simulink model "mchp_acim_dsPIC33A"  (R2025b)
settings: Solver=FixedStepDiscrete  StartTime=0.0  StopTime=25  FixedStep=Ts  RelTol=1e-3  EnableMultiTasking=on
values from neighbouring files (symbols this model uses):
  dataType = 'single'    [mchp_acim_foc_dsPIC33A_data.m]
  PWM_frequency = 20e3    (= 20000)    [mchp_acim_foc_dsPIC33A_data.m]
  PWM_frequency_mc = PWM_frequency    (= 20000)    [mchp_acim_foc_dsPIC33A_data.m]
  SpeedFilterCutoff = 40    [mchp_acim_foc_dsPIC33A_data.m]
  Ts = T_pwm    (= 5e-05)    [mchp_acim_foc_dsPIC33A_data.m]
  Ts_mc = T_pwm_mc    (= 5e-05)    [mchp_acim_foc_dsPIC33A_data.m]
  Ts_motor = T_pwm_mc    (= 5e-05)    [mchp_acim_foc_dsPIC33A_data.m]
  Ts_serialIn = 100e-3    (= 0.1)    [mchp_acim_foc_dsPIC33A_data.m]
undefined symbols (not defined in the file or in its folder): A0, A4, acim, ADC, appState, B0, C10, C11, C6, C7, C8, CS_param, D11, D12, DiscIntNeverNeededParam, estim_pll, estim_qei, inverter, Max, MaxPer, ms, NumBits1, NumBits2, P1, P17, P20, P39, P40, P41, P43, P44, P60, P61, PI_params_SI, Pin, PWM4_Trg1, Resol, s, target, us, VmaxPhase
libraries: simulink x47, MCHP_Blockset x24, mcbcontrolslib x5, mcbeeMathTransformLib x4, slpidlib x4, svdutilitieslib x1, autolibim x1, mcbplantlib x1
(part 3 of 6)

== system mchp_acim_dsPIC33A/Subsystem ==
  Control mode : Constant  OutDataTypeStr=single
  DC bus compensation : Constant  OutDataTypeStr=single  SampleTime=-1
  Data Store Write : DataStoreWrite  DataStoreName=ControlMode  IndexOptions=Index vector (dialog)  Indices=1  OutputSizes=1
  Data Store Write1 : DataStoreWrite  DataStoreName=FluxWeakeningOperation  IndexOptions=Index vector (dialog)  Indices=1  OutputSizes=1
  Data Store Write2 : DataStoreWrite  DataStoreName=DC_BusCompensation  IndexOptions=Index vector (dialog)  Indices=1  OutputSizes=1
  Flux weakening operation : Constant  OutDataTypeStr=single  SampleTime=-1
  wires:
  Control mode/1 -> Data Store Write/1
  Flux weakening operation/1 -> Data Store Write1/1
  DC bus compensation/1 -> Data Store Write2/1

== system mchp_acim_dsPIC33A/Control algorithm/Application_Abstraction ==
  Iab_Measured : Inport
  position_count : Inport  Port=2
  Bias : Bias  Bias=-1  SaturateOnIntegerOverflow=off
  Bus Creator : BusCreator  Inputs=1
  Constant2 : Constant  OutDataTypeStr=single  SampleTime=-1
  Gain2 : Gain  Gain=(2/(acim.QEPSlits*4))  ParamDataTypeStr=single  OutDataTypeStr=single
  Subsystem1 : Subsystem
  Currents : Outport
  RotorSpeed : Outport  Port=2
  wires:
  Iab_Measured/1 -> Bus Creator/1  "Iab"
  Bus Creator/1 -> Currents/1
  Gain2/1 -> Bias/1
  Constant2/1 -> Subsystem1/2(Enable)
  position_count/1 -> Gain2/1
  Subsystem1/1(speed_mech_rpm) -> RotorSpeed/1  "omegaRotorRPM"
  Bias/1 -> Subsystem1/1(thetaMech_PU)

== system mchp_acim_dsPIC33A/Control algorithm/Command_Signals ==
  note: Subsystem
  Command_Data : Inport
  Add : Sum
  Bus Creator : BusCreator  Inputs=2
  Constant : Constant  Value=acim.N_min  OutDataTypeStr=single  SampleTime=-1
  Constant1 : Constant  Value=acim.N_max  OutDataTypeStr=single  SampleTime=-1
  Constant2 : Constant  Value=acim.N_min  OutDataTypeStr=single  SampleTime=-1
  Data Type Conversion1 : DataTypeConversion  OutDataTypeStr=single  RndMeth=Simplest  SaturateOnIntegerOverflow=off
  Data Type Conversion4 : DataTypeConversion  OutDataTypeStr=single  RndMeth=Simplest  SaturateOnIntegerOverflow=off
  Demux : Demux  Outputs=2
  Gain2 : Gain
  Product : Product
  Rate Limiter2 : RateLimiter  RisingSlewLimit=0.2  FallingSlewLimit=-0.2  SampleTimeMode=inherited
  Subtract : Sum  Inputs=+-
  Triggered Subsystem : Subsystem  TreatAsAtomicUnit=on
  Commands : Outport
  wires:
  Bus Creator/1 -> Commands/1
  Data Type Conversion1/1 -> Bus Creator/1  "RunCmd"
  Data Type Conversion4/1 -> Bus Creator/2  "TargetSpeed"
  Gain2/1 -> Data Type Conversion4/1
  Product/1 -> Add/2
  Demux/2 -> Rate Limiter2/1
  Constant/1 -> Subtract/2
  Subtract/1 -> Product/2
  Add/1 -> Gain2/1
  Command_Data/1 -> Demux/1
  Triggered Subsystem/1(RunCmd) -> Data Type Conversion1/1
  Constant2/1 -> Add/1
  Demux/1 -> Triggered Subsystem/Trigger
  Constant1/1 -> Subtract/1
  Rate Limiter2/1 -> Product/1

== system mchp_acim_dsPIC33A/Control algorithm/Command_Signals_simulation ==
  Add : Sum
  Add1 : Sum  Inputs=+++
  Bus Creator : BusCreator  Inputs=2
  Constant : Constant  Value=acim.N_min  OutDataTypeStr=single  SampleTime=-1
  Constant1 : Constant  Value=acim.N_max  OutDataTypeStr=single  SampleTime=-1
  Constant2 : Constant  Value=acim.N_min  OutDataTypeStr=single  SampleTime=-1
  Data Type Conversion2 : DataTypeConversion  OutDataTypeStr=single  RndMeth=Simplest  SaturateOnIntegerOverflow=off
  Product : Product
  Rate Limiter2 : RateLimiter  RisingSlewLimit=0.2  FallingSlewLimit=-0.2  SampleTimeMode=inherited
  Step : Step  Time=0  OutDataTypeStr=single  SampleTime=Ts_mc
  Step1 : Step  Time=20  After=-1  OutDataTypeStr=single  SampleTime=Ts_mc
  Step2 : Step  Time=30  After=2  OutDataTypeStr=single  SampleTime=Ts_mc
  Step4 : Step  OutDataTypeStr=single  SampleTime=Ts_mc
  Subtract : Sum  Inputs=+-
  Commands : Outport
  wires:
  Bus Creator/1 -> Commands/1
  Data Type Conversion2/1 -> Bus Creator/1  "RunCmd"
  Add/1 -> Bus Creator/2  "TargetSpeed"
  Product/1 -> Add/2
  Step4/1 -> Add1/1
  Constant1/1 -> Subtract/1
  Constant2/1 -> Add/1
  Subtract/1 -> Product/2
  Step/1 -> Rate Limiter2/1
  Constant/1 -> Subtract/2
  Add1/1 -> Data Type Conversion2/1
  Step1/1 -> Add1/2
  Step2/1 -> Add1/3
  Rate Limiter2/1 -> Product/1

== system mchp_acim_dsPIC33A/Control algorithm/Data Monitoring ==
  Data_Monitor : Inport
  Constant : Constant  OutDataTypeStr=boolean
  Rate Transition13 : RateTransition  Deterministic=off  OutPortSampleTime=Ts_serialIn
  Rate Transition14 : RateTransition  Deterministic=off  OutPortSampleTime=Ts_serialOut
  Rate Transition15 : RateTransition  Deterministic=off  OutPortSampleTime=Ts_serialOut
  SerialInDrivers : Subsystem
  SerialOutDrivers : Subsystem  Variant=on  VariantControlMode=sim codegen switching
  Subsystem : Subsystem
  Terminator : Terminator
  Variant Subsystem : Subsystem  Variant=on  VariantControlMode=sim codegen switching
  wires:
  Variant Subsystem/1(ConfigAndCommand) -> Terminator/1
  Constant/1 -> Rate Transition13/1
  Rate Transition15/1 -> Subsystem/1(DebugSel)
  Rate Transition14/1 -> Subsystem/2(DebugData)
  Variant Subsystem/2(DebugSel) -> Rate Transition15/1
  Rate Transition13/1 -> Variant Subsystem/2(Mode)
  Subsystem/1(Debug_signal) -> SerialOutDrivers/1(SerialData)
  SerialInDrivers/1(SCI_Data) -> Variant Subsystem/1(SCI_Data)  "sci data 8 bytes"
  Data_Monitor/1 -> Rate Transition14/1

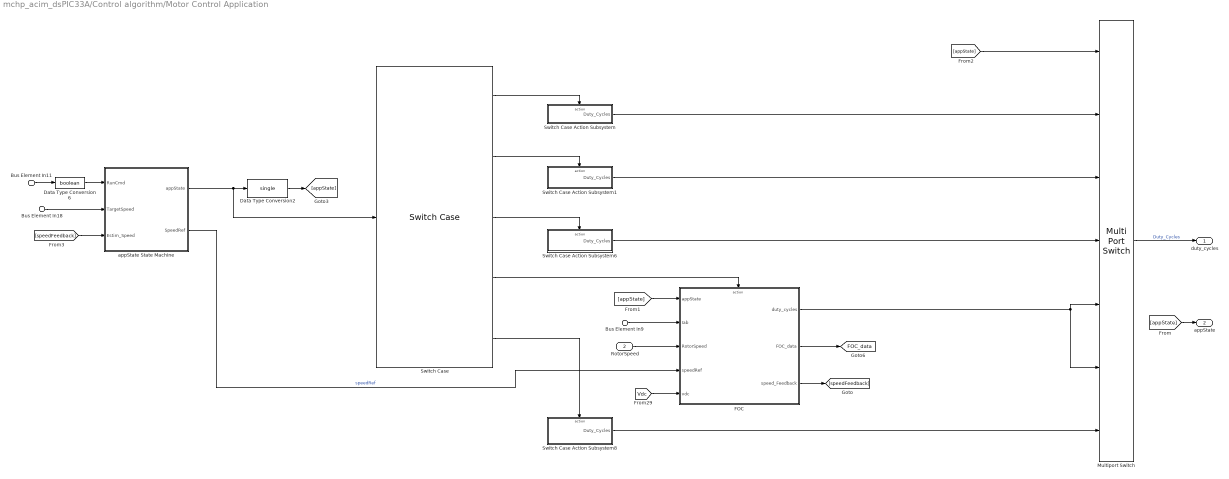
== system mchp_acim_dsPIC33A/Control algorithm/Motor Control Application ==
  Bus Element In9 : Inport  PortName=Currents  Element=Iab
  RotorSpeed : Inport  Port=2
  Bus Element In11 : Inport  Port=3  PortName=Commands  Element=RunCmd
  Bus Element In18 : Inport  Port=3  PortName=Commands  Element=TargetSpeed
  Data Type Conversion2 : DataTypeConversion  OutDataTypeStr=single  SaturateOnIntegerOverflow=off  RndMeth=Floor
  Data Type Conversion6 : DataTypeConversion  OutDataTypeStr=boolean  SaturateOnIntegerOverflow=off  RndMeth=Floor
  FOC : Subsystem  TreatAsAtomicUnit=on
  Multiport Switch : MultiPortSwitch  DataPortOrder=Zero-based contiguous  Inputs=6  zeroidx=on  SaturateOnIntegerOverflow=off  InputSameDT=off
  Switch Case : SwitchCase  CaseConditions={appState.INIT,appState.OFFSET_MEAS,appState.CMD_WAIT,[appState.VF_OPEN_LOOP,appState.FOC_CLOSED_LOOP], appState.STOP}  ShowDefaultCase=off
  Switch Case Action Subsystem : Subsystem  TreatAsAtomicUnit=on
  Switch Case Action Subsystem1 : Subsystem  TreatAsAtomicUnit=on
  Switch Case Action Subsystem6 : Subsystem  TreatAsAtomicUnit=on
  Switch Case Action Subsystem8 : Subsystem  TreatAsAtomicUnit=on
  appState State Machine : Subsystem
  duty_cycles : Outport  VectorParamsAs1DForOutWhenUnconnected=off
  appState : Outport  Port=2  VectorParamsAs1DForOutWhenUnconnected=off
  tag scope: FOC_data=global
  wires:
  appState State Machine/2(SpeedRef) -> FOC/4(speedRef)  "speedRef"
  Multiport Switch/1 -> duty_cycles/1  "Duty_Cycles"
  Switch Case/3 -> Switch Case Action Subsystem6/Action
  Switch Case Action Subsystem/1(Duty_Cycles) -> Multiport Switch/2
  [appState] -> Multiport Switch/1
  Bus Element In11/1 -> Data Type Conversion6/1
  Switch Case/4 -> FOC/Action
  Switch Case/1 -> Switch Case Action Subsystem/Action
  Switch Case/5 -> Switch Case Action Subsystem8/Action
  Switch Case Action Subsystem1/1(Duty_Cycles) -> Multiport Switch/3
  Switch Case Action Subsystem6/1(Duty_Cycles) -> Multiport Switch/4
  Data Type Conversion6/1 -> appState State Machine/1(RunCmd)
  Switch Case Action Subsystem8/1(Duty_Cycles) -> Multiport Switch/7
  Switch Case/2 -> Switch Case Action Subsystem1/Action
  appState State Machine/1(appState) -> Switch Case/1, Data Type Conversion2/1
  Bus Element In9/1 -> FOC/2(Iab)
  FOC/1(duty_cycles) -> Multiport Switch/6, Multiport Switch/5
  Data Type Conversion2/1 -> [appState]
  RotorSpeed/1 -> FOC/3(RotorSpeed)
  FOC/2(FOC_data) -> [FOC_data]
  [appState] -> FOC/1(appState)
  [appState] -> appState/1
  Bus Element In18/1 -> appState State Machine/2(TargetSpeed)
  [Vdc] -> FOC/5(vdc)
  FOC/3(speed_Feedback) -> [speedFeedback]
  [speedFeedback] -> appState State Machine/3(Estim_Speed)

== system mchp_acim_dsPIC33A/Inverter and Motor model/Codegeneration ==
  Duty_Cycles : Inport
  Ground : Ground
  Terminator : Terminator
  Feedbacks : Outport  VectorParamsAs1DForOutWhenUnconnected=off
  wires:
  Duty_Cycles/1 -> Terminator/1
  Ground/1 -> Feedbacks/1

== system mchp_acim_dsPIC33A/Inverter and Motor model/Simulation ==
  Duty_Cycles : Inport
  Load_Profile (Torque) : Subsystem
  Motor and Inverter : Subsystem  VariantControl=(get_param([bdroot '/InverterSelected'], 'Value') == '0')
  RT1 : RateTransition  Deterministic=off  OutPortSampleTime=Ts_simulink
  RT3 : RateTransition  Deterministic=off  OutPortSampleTime=Ts_simulink
  Sensor_Measurements : Subsystem
  Feedbacks : Outport  VectorParamsAs1DForOutWhenUnconnected=off
  wires:
  Sensor_Measurements/1(Sim_fb) -> Feedbacks/1
  Load_Profile (Torque)/1(Load_Trq) -> Motor and Inverter/2(Load)
  Motor and Inverter/1(Iabc) -> RT1/1  "Iabc"
  Duty_Cycles/1 -> Motor and Inverter/1(Vabc_In_PU)
  RT3/1 -> Sensor_Measurements/2(pos)
  Motor and Inverter/2(Theta) -> RT3/1
  RT1/1 -> Sensor_Measurements/1(PhaseCurr)
